simulink subsystem "Spline_Steering_and_Drive_Commands"  (R2023b)
settings: Solver=VariableStepAuto  StartTime=0.0  StopTime=10.0  RelTol=1e-3
settings Model: Creator=ander  LastModifiedBy=ander

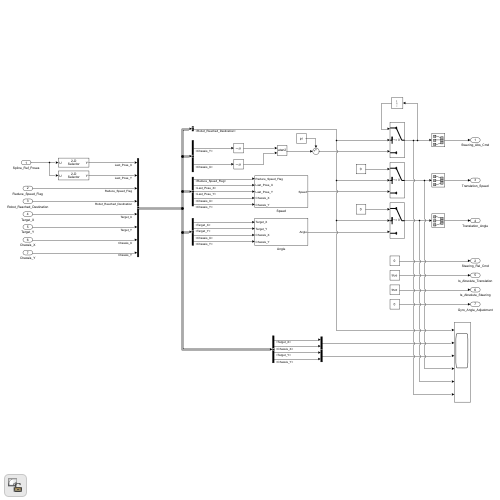
[thumbnail: Simulink's stored preview of the top-level diagram]
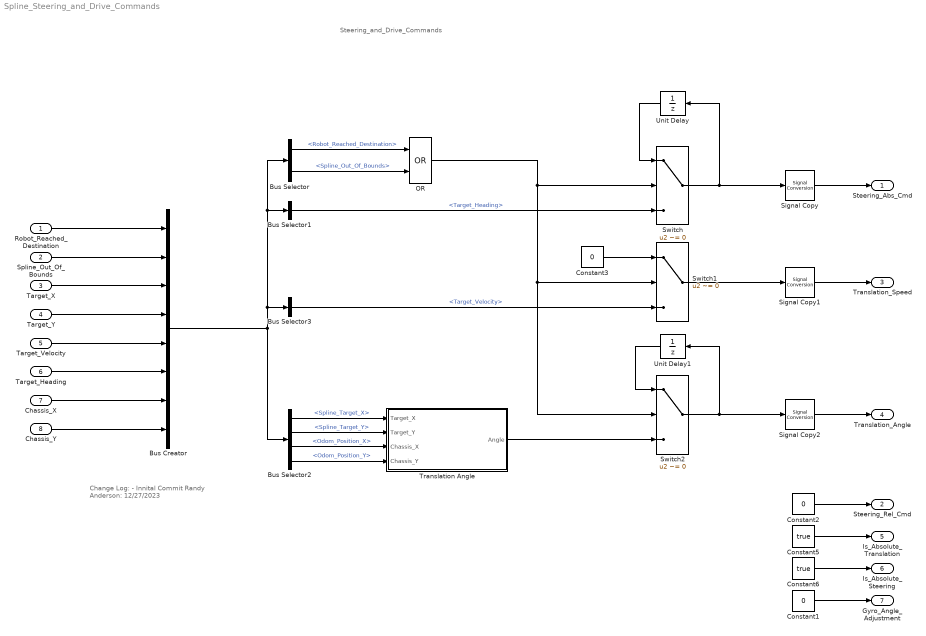
== system Spline_Steering_and_Drive_Commands ==
  note: Steering_and_Drive_Commands
  note: Change Log:
      | - Innital Commit
      | Randy Anderson: 12/27/2023
  Robot_Reached_Destination : Inport
  Spline_Out_Of_Bounds : Inport  Port=2
  Target_X : Inport  Port=3
  Target_Y : Inport  Port=4
  Target_Velocity : Inport  Port=5
  Target_Heading : Inport  Port=6
  Chassis_X : Inport  Port=7  OutDataTypeStr=double  PortDimensions=1
  Chassis_Y : Inport  Port=8  OutDataTypeStr=double  PortDimensions=1
  Bus Creator : BusCreator  Inputs=8
  Bus Selector : BusSelector  OutputSignals=Robot_Reached_Destination,Spline_Out_Of_Bounds
  Bus Selector1 : BusSelector  OutputSignals=Target_Heading
  Bus Selector2 : BusSelector  OutputSignals=Spline_Target_X,Spline_Target_Y,Odom_Position_X,Odom_Position_Y
  Bus Selector3 : BusSelector  OutputSignals=Target_Velocity
  Constant1 : Constant  Value=0
  Constant2 : Constant  Value=0
  Constant3 : Constant  Value=0
  Constant5 : Constant  Value=true
  Constant6 : Constant  Value=true
  OR : Logic  Operator=OR  AllPortsSameDT=off  OutDataTypeStr=boolean
  Signal Copy : SignalConversion  OverrideOpt=off
  Signal Copy1 : SignalConversion  OverrideOpt=off
  Signal Copy2 : SignalConversion  OverrideOpt=off
  Switch : Switch  Criteria=u2 ~= 0  SaturateOnIntegerOverflow=off  InputSameDT=off
  Switch1 : Switch  Criteria=u2 ~= 0  SaturateOnIntegerOverflow=off  InputSameDT=off
  Switch2 : Switch  Criteria=u2 ~= 0  SaturateOnIntegerOverflow=off  InputSameDT=off
  Translation Angle : Subsystem
  Unit Delay : UnitDelay  SampleTime=-1  HasFrameUpgradeWarning=on
  Unit Delay1 : UnitDelay  SampleTime=-1  HasFrameUpgradeWarning=on
  Steering_Abs_Cmd : Outport
  Steering_Rel_Cmd : Outport  Port=2
  Translation_Speed : Outport  Port=3
  Translation_Angle : Outport  Port=4
  Is_Absolute_Translation : Outport  Port=5
  Is_Absolute_Steering : Outport  Port=6
  Gyro_Angle_Adjustment : Outport  Port=7
  wires:
  Constant1/1 -> Gyro_Angle_Adjustment/1
  Constant5/1 -> Is_Absolute_Translation/1
  Constant6/1 -> Is_Absolute_Steering/1
  Constant2/1 -> Steering_Rel_Cmd/1
  Switch/1 -> Unit Delay/1, Signal Copy/1
  Bus Selector1/1 -> Switch/3  "<Target_Heading>"
  Switch1/1 -> Signal Copy1/1
  Switch2/1 -> Signal Copy2/1, Unit Delay1/1
  OR/1 -> Switch/2, Switch1/2, Switch2/2
  Constant3/1 -> Switch1/1
  Unit Delay/1 -> Switch/1
  Signal Copy/1 -> Steering_Abs_Cmd/1
  Signal Copy1/1 -> Translation_Speed/1
  Signal Copy2/1 -> Translation_Angle/1
  Bus Creator/1 -> Bus Selector1/1, Bus Selector/1, Bus Selector3/1, Bus Selector2/1
  Translation Angle/1(Angle) -> Switch2/3
  Bus Selector2/1 -> Translation Angle/1(Target_X)  "<Spline_Target_X>"
  Bus Selector2/2 -> Translation Angle/2(Target_Y)  "<Spline_Target_Y>"
  Bus Selector2/3 -> Translation Angle/3(Chassis_X)  "<Odom_Position_X>"
  Bus Selector2/4 -> Translation Angle/4(Chassis_Y)  "<Odom_Position_Y>"
  Robot_Reached_Destination/1 -> Bus Creator/1
  Bus Selector3/1 -> Switch1/3  "<Target_Velocity>"
  Unit Delay1/1 -> Switch2/1
  Spline_Out_Of_Bounds/1 -> Bus Creator/2
  Target_X/1 -> Bus Creator/3
  Target_Y/1 -> Bus Creator/4
  Target_Velocity/1 -> Bus Creator/5
  Target_Heading/1 -> Bus Creator/6
  Chassis_X/1 -> Bus Creator/7
  Chassis_Y/1 -> Bus Creator/8
  Bus Selector/1 -> OR/1  "<Robot_Reached_Destination>"
  Bus Selector/2 -> OR/2  "<Spline_Out_Of_Bounds>"

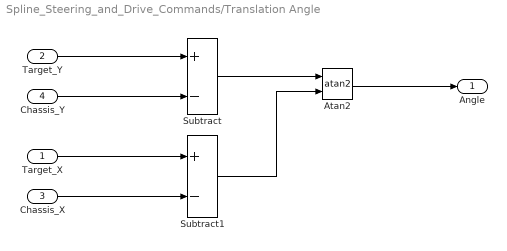
== system Spline_Steering_and_Drive_Commands/Translation Angle ==
  Target_X : Inport
  Target_Y : Inport  Port=2
  Chassis_X : Inport  Port=3
  Chassis_Y : Inport  Port=4
  Atan2 : Trigonometry  Operator=atan2
  Subtract : Sum  Inputs=+-
  Subtract1 : Sum  Inputs=+-
  Angle : Outport
  wires:
  Chassis_Y/1 -> Subtract/2
  Target_Y/1 -> Subtract/1
  Atan2/1 -> Angle/1
  Subtract/1 -> Atan2/1
  Target_X/1 -> Subtract1/1
  Chassis_X/1 -> Subtract1/2
  Subtract1/1 -> Atan2/2
